simulink model "Simulink_Simulink_PIL_Cruise_Crontrol_r2020b"  (R2024a)
settings: Solver=VariableStepAuto  StartTime=0.0  StopTime=Tsim  FixedStep=Ts/20  RelTol=1e-3
undefined symbols (not defined in the file or in its folder): g, noise, PIL, Ts
libraries: simulink x2, aerolibactuator x1, aerolibatmos2 x1
settings Model: SimulationMode=accelerator  Creator=ricardo  LastModifiedBy=mason
settings SolverCC: AlgebraicLoopSolver=TrustRegion
settings DataIOCC: ReturnWorkspaceOutputs=off
settings DebuggingCC: UnconnectedInputMsg=warning  UnconnectedOutputMsg=warning  UnconnectedLineMsg=warning  ArithmeticOperatorsInVariantConditions=warning
settings ModelReferenceCC: EnableRefExpFcnMdlSchedulingChecks=on
settings SFSimCC: CustomCodeUndefinedFunction=UseInterfaceOnly
settings RTWCC: GPUComputeCapability=3.5  DLArmComputeVersion=19.05

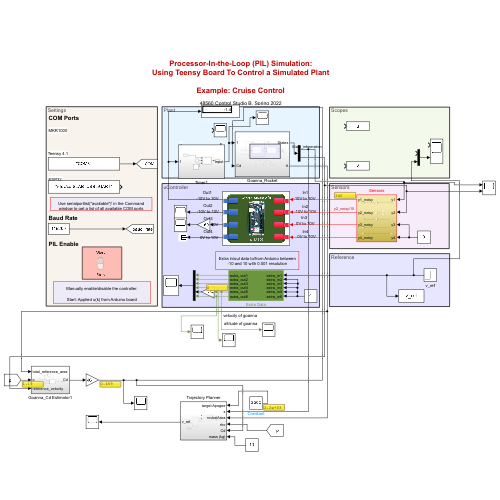
[thumbnail: Simulink's stored preview of the top-level diagram]
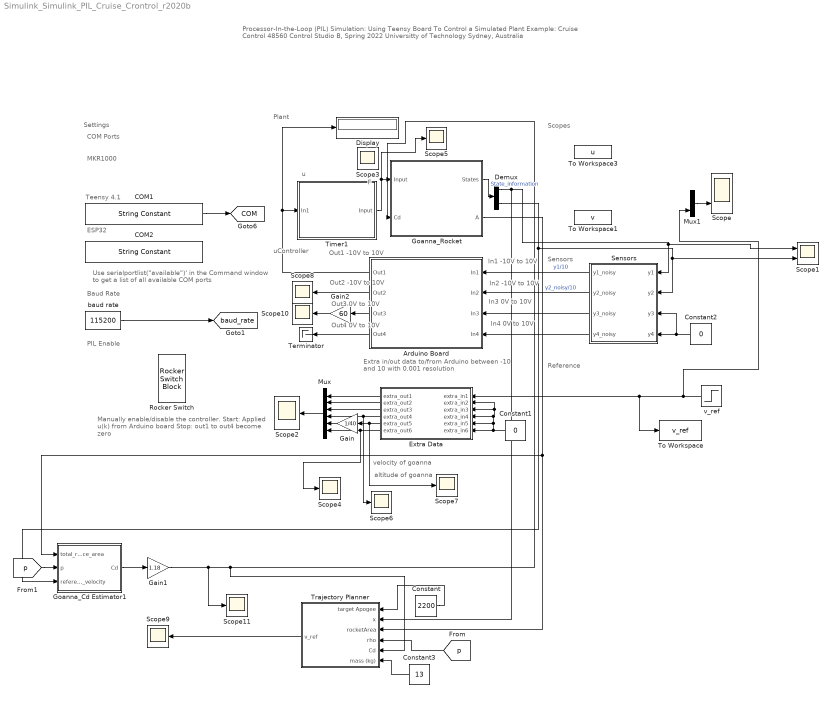
== system Simulink_Simulink_PIL_Cruise_Crontrol_r2020b ==
  note: altitude of goanna
  note: velocity of goanna
  note: F
  note: u
  note: MKR1000
  note: COM Ports
  note: Settings
  note: Scopes
  note: Plant
  note: Reference
  note: Sensors
  note: uController
  note: Out1
      | -10V to 10V
  note: Processor-In-the-Loop (PIL) Simulation:
      | Using Teensy Board To Control a Simulated Plant
      |
      | Example: Cruise Control
      |
      | 48560 Control Studio B, Spring 2022
      | Universitty of Technology Sydney, Australia
  note: Out2
      | -10V to 10V
  note: Out3
      | 0V to 10V
  note: Out4
      | 0V to 10V
  note: In1
      | -10V to 10V
  note: In2
      | -10V to 10V
  note: In3
      | 0V to 10V
  note: In4
      | 0V to 10V
  note: Manually enable/disable the controller.
      |
      | Start: Applied u(k) from Arduino board
      | Stop: out1 to out4 become zero
  note: Extra in/out data to/from Arduino between -10 and 10 with 0.001 resolution
  note: Baud Rate
  note: PIL Enable
  note: Use serialportlist("available")' in the Command window to get a list of all available COM ports
  note: ESP32
  note: Teensy 4.1
  Arduino Board : Subsystem
      mask Display: image('$imagefile'); % Use "Edit Image" on toolstrip to change.
  COM1 : StringConstant  String="\"COM8\""
  COM2 : StringConstant  String="\"/dev/cu.SLAB_USBtoUART\""
  Constant : Constant  Value=2200
  Constant1 : Constant  Value=0
  Constant2 : Constant  Value=0
  Constant3 : Constant  Value=13
  Demux : Demux  Outputs=2
  Display : Display
  Extra Data : Subsystem
  Gain : Gain  Gain=1/40
  Gain1 : Gain  Gain=1.18
  Gain2 : Gain  Gain=60
  Goanna_Cd Estimator1 : Subsystem
  Goanna_Rocket : Subsystem
  Mux : Mux  Inputs=6
  Mux1 : Mux  Inputs=2
  Rocker Switch : RockerSwitchBlock  LabelPosition=Hide
      settings: Values={{'Stop', 'Start'}, [0 1]}
  Scope : Scope  NumInputPorts=2
  Scope1 : Scope  NumInputPorts=2
  Scope{2..11} (10 alike) : Scope
  Sensors : Subsystem
  Terminator : Terminator
  Timer1 : Subsystem
  To Workspace : ToWorkspace  VariableName=v_ref  SampleTime=Ts/20
  To Workspace1 : ToWorkspace  VariableName=v  SampleTime=Ts/20
  To Workspace3 : ToWorkspace  VariableName=u  SampleTime=Ts/20
  Trajectory Planner : Subsystem
  baud rate : Constant  Value=115200
  v_ref : Step  Time=5  After=5  SampleTime=0
  tag scope: COM=global, baud_rate=global
  wires:
  Arduino Board/2(Out2) -> Scope8/1
  Arduino Board/3(Out3) -> Gain2/1
  Arduino Board/4(Out4) -> Terminator/1
  Extra Data/1(extra_out1) -> Mux/1
  Extra Data/2(extra_out2) -> Mux/2
  Extra Data/3(extra_out3) -> Mux/3
  Extra Data/4(extra_out4) -> Scope6/1, Mux/4
  Mux/1 -> Scope2/1
  Extra Data/5(extra_out5) -> Gain/1, Scope7/1
  Extra Data/6(extra_out6) -> Scope4/1, Mux/6
  Constant1/1 -> Extra Data/2(extra_in2), Extra Data/3(extra_in3), Extra Data/4(extra_in4), Extra Data/5(extra_in5), Extra Data/6(extra_in6)
  Sensors/1(y1_noisy) -> Arduino Board/1(In1)  "y1/10"
  Constant2/1 -> Sensors/3(y3), Sensors/4(y4)
  Sensors/4(y4_noisy) -> Arduino Board/4(In4)
  baud rate/1 -> [baud_rate]
  Sensors/2(y2_noisy) -> Arduino Board/2(In2)  "y2_noisy/10"
  Sensors/3(y3_noisy) -> Arduino Board/3(In3)
  v_ref/1 -> Extra Data/1(extra_in1), To Workspace/1, Mux1/2
  Mux1/1 -> Scope/2
  COM1/1 -> [COM]
  Goanna_Rocket/1(States) -> Demux/1  "State_information"
  Demux/1 -> Scope1/1, Sensors/1(y1), Trajectory Planner/2(x)
  Demux/2 -> Goanna_Cd Estimator1/3(reference_velocity), Scope1/2, Sensors/2(y2)
  Goanna_Cd Estimator1/1(Cd) -> Gain1/1
  Gain/1 -> Mux/5
  Gain1/1 -> Scope11/1, Trajectory Planner/5(Cd), Goanna_Rocket/2(Cd)
  Goanna_Rocket/2(A) -> Trajectory Planner/3(rocketArea), Goanna_Cd Estimator1/1(total_reference_area)
  Constant/1 -> Trajectory Planner/1(target Apogee)
  [p] -> Trajectory Planner/4(rho)
  Constant3/1 -> Trajectory Planner/6(mass (kg))
  [p] -> Goanna_Cd Estimator1/2(p)
  Trajectory Planner/1(v_ref) -> Scope9/1
  Gain2/1 -> Scope10/1
  Timer1/1(Input) -> Scope5/1, Goanna_Rocket/1(Input)
  Arduino Board/1(Out1) -> Display/1, Timer1/1(In1)

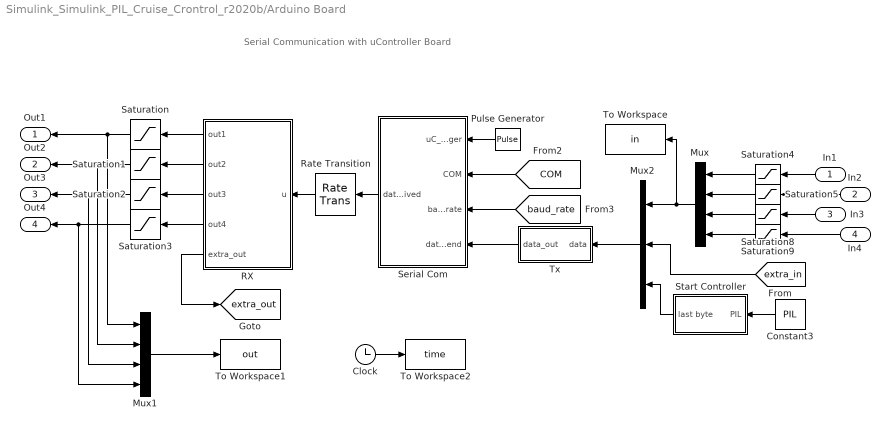
== system Simulink_Simulink_PIL_Cruise_Crontrol_r2020b/Arduino Board ==
  note: Serial Communication with uController Board
  In1 : Inport
  In2 : Inport  Port=2
  In3 : Inport  Port=3
  In4 : Inport  Port=4
  Clock : Clock
  Constant3 : Constant  Value=PIL
  Mux : Mux
  Mux1 : Mux
  Mux2 : Mux  Inputs=3
  Pulse Generator : DiscretePulseGenerator  PulseType=Time based  Period=Ts  PulseWidth=50
  RX : MATLAB Function  TreatAsAtomicUnit=on
  Rate Transition : RateTransition  InitialCondition=zeros(21,1)
  Saturation{,1,4..5} (4 alike) : Saturate  UpperLimit=10  LowerLimit=-10
  Saturation{2..3,8..9} (4 alike) : Saturate  UpperLimit=10  LowerLimit=0
  Serial Com : MATLAB Function  TreatAsAtomicUnit=on  SystemSampleTime=Ts/10
  Start Controller : Subsystem
  To Workspace : ToWorkspace  VariableName=in  SampleTime=Ts/20
  To Workspace1 : ToWorkspace  VariableName=out  SampleTime=Ts/20
  To Workspace2 : ToWorkspace  VariableName=time  SampleTime=Ts/20
  Tx : MATLAB Function  TreatAsAtomicUnit=on  SystemSampleTime=Ts/10
  Out1 : Outport  VectorParamsAs1DForOutWhenUnconnected=off
  Out2 : Outport  Port=2  VectorParamsAs1DForOutWhenUnconnected=off
  Out3 : Outport  Port=3  VectorParamsAs1DForOutWhenUnconnected=off
  Out4 : Outport  Port=4  VectorParamsAs1DForOutWhenUnconnected=off
  tag scope: extra_out=global
  wires:
  RX/1(out1) -> Saturation/1
  RX/2(out2) -> Saturation1/1
  RX/3(out3) -> Saturation2/1
  Mux1/1 -> To Workspace1/1
  Clock/1 -> To Workspace2/1
  Saturation/1 -> Out1/1, Mux1/1
  Saturation1/1 -> Out2/1, Mux1/2
  Saturation2/1 -> Out3/1, Mux1/3
  Saturation3/1 -> Out4/1, Mux1/4
  RX/4(out4) -> Saturation3/1
  RX/5(extra_out) -> [extra_out]
  Mux/1 -> Mux2/1, To Workspace/1
  [COM] -> Serial Com/2(COM)
  [baud_rate] -> Serial Com/3(baud_rate)
  Pulse Generator/1 -> Serial Com/1(uC_trigger)
  Serial Com/1(data_received) -> Rate Transition/1
  Rate Transition/1 -> RX/1(u)
  Constant3/1 -> Start Controller/1(PIL)
  In1/1 -> Saturation4/1
  In2/1 -> Saturation5/1
  In3/1 -> Saturation8/1
  In4/1 -> Saturation9/1
  Saturation4/1 -> Mux/1
  Saturation5/1 -> Mux/2
  Saturation8/1 -> Mux/3
  Saturation9/1 -> Mux/4
  [extra_in] -> Mux2/2
  Start Controller/1(last byte) -> Mux2/3
  Mux2/1 -> Tx/1(data)
  Tx/1(data_out) -> Serial Com/4(data_send)

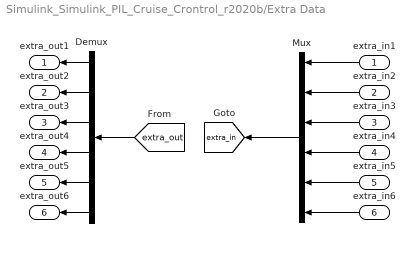
== system Simulink_Simulink_PIL_Cruise_Crontrol_r2020b/Extra Data ==
  extra_in1 : Inport
  extra_in2 : Inport  Port=2
  extra_in3 : Inport  Port=3
  extra_in4 : Inport  Port=4
  extra_in5 : Inport  Port=5
  extra_in6 : Inport  Port=6
  Demux : Demux  Outputs=6
  Mux : Mux  Inputs=6
  extra_out1 : Outport
  extra_out2 : Outport  Port=2
  extra_out3 : Outport  Port=3
  extra_out4 : Outport  Port=4
  extra_out5 : Outport  Port=5
  extra_out6 : Outport  Port=6
  tag scope: extra_in=global
  wires:
  extra_in4/1 -> Mux/4
  extra_in3/1 -> Mux/3
  extra_in2/1 -> Mux/2
  extra_in1/1 -> Mux/1
  Mux/1 -> [extra_in]
  [extra_out] -> Demux/1
  Demux/1 -> extra_out1/1
  Demux/2 -> extra_out2/1
  Demux/3 -> extra_out3/1
  Demux/4 -> extra_out4/1
  extra_in5/1 -> Mux/5
  extra_in6/1 -> Mux/6
  Demux/6 -> extra_out6/1
  Demux/5 -> extra_out5/1

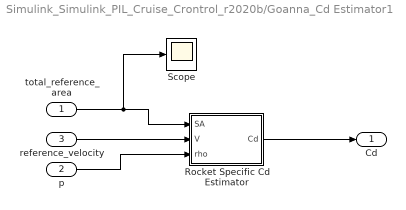
== system Simulink_Simulink_PIL_Cruise_Crontrol_r2020b/Goanna_Cd Estimator1 ==
  total_reference_area : Inport
  p : Inport  Port=2
  reference_velocity : Inport  Port=3
  Rocket Specific Cd Estimator : MATLAB Function  TreatAsAtomicUnit=on
  Scope : Scope
  Cd : Outport
  wires:
  Rocket Specific Cd Estimator/1(Cd) -> Cd/1
  total_reference_area/1 -> Scope/1, Rocket Specific Cd Estimator/1(SA)
  reference_velocity/1 -> Rocket Specific Cd Estimator/2(V)
  p/1 -> Rocket Specific Cd Estimator/3(rho)

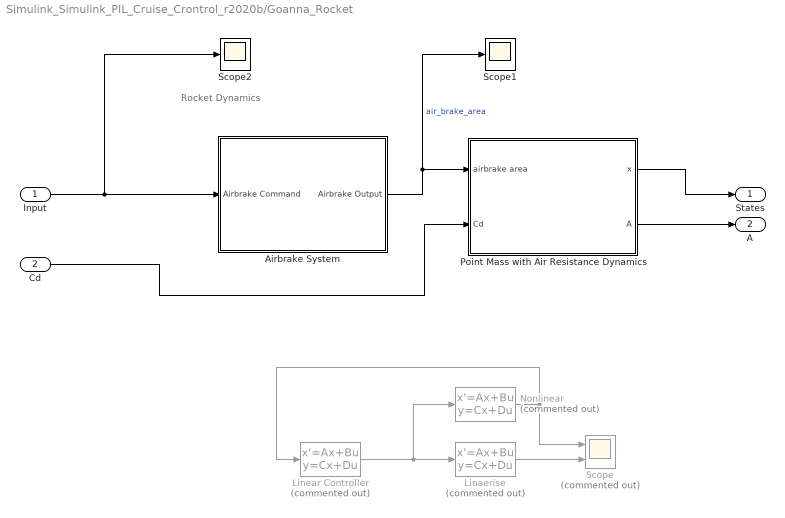
== system Simulink_Simulink_PIL_Cruise_Crontrol_r2020b/Goanna_Rocket ==
  note: Rocket Dynamics
  Input : Inport
  Cd : Inport  Port=2
  Airbrake System : Subsystem
      mask Display: image('airbrake.png');
  "Linaerise " : StateSpace  Commented=on  InitialCondition=0
  Linear Controller : StateSpace  Commented=on  InitialCondition=0
  Nonlinear : StateSpace  Commented=on  InitialCondition=0
  "Point Mass with Air Resistance Dynamics " : Subsystem
      mask Display: image('rocket.jpeg');
  Scope : Scope  Commented=on  NumInputPorts=2
  Scope1 : Scope
  Scope2 : Scope
  States : Outport
  A : Outport  Port=2
  wires:
  "Point Mass with Air Resistance Dynamics "/1(x) -> States/1
  Linear Controller/1 -> Nonlinear/1, "Linaerise "/1
  Nonlinear/1 -> Linear Controller/1, Scope/1
  "Linaerise "/1 -> Scope/2
  Input/1 -> Scope2/1, Airbrake System/1(Airbrake Command)
  Airbrake System/1(Airbrake Output) -> "Point Mass with Air Resistance Dynamics "/1(airbrake area), Scope1/1  "air_brake_area"
  Cd/1 -> "Point Mass with Air Resistance Dynamics "/2(Cd)
  "Point Mass with Air Resistance Dynamics "/2(A) -> A/1

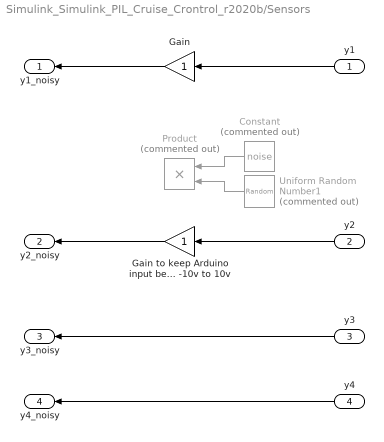
== system Simulink_Simulink_PIL_Cruise_Crontrol_r2020b/Sensors ==
  y1 : Inport
  y2 : Inport  Port=2
  y3 : Inport  Port=3
  y4 : Inport  Port=4
  Constant : Constant  Commented=on  Value=noise
  Gain : Gain
  "Gain to keep Arduino input between -10v to 10v " : Gain
  Product : Product  Commented=on
  Uniform Random Number1 : UniformRandomNumber  Commented=on  Minimum=-0.1  Maximum=0.1  SampleTime=0.5*Ts
  y1_noisy : Outport  VectorParamsAs1DForOutWhenUnconnected=off
  y2_noisy : Outport  Port=2  VectorParamsAs1DForOutWhenUnconnected=off
  y3_noisy : Outport  Port=3  VectorParamsAs1DForOutWhenUnconnected=off
  y4_noisy : Outport  Port=4  VectorParamsAs1DForOutWhenUnconnected=off
  wires:
  y2/1 -> "Gain to keep Arduino input between -10v to 10v "/1
  y3/1 -> y3_noisy/1
  y4/1 -> y4_noisy/1
  y1/1 -> Gain/1
  Uniform Random Number1/1 -> Product/2
  Constant/1 -> Product/1
  "Gain to keep Arduino input between -10v to 10v "/1 -> y2_noisy/1
  Gain/1 -> y1_noisy/1

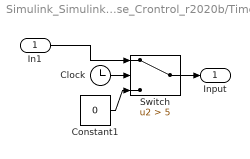
== system Simulink_Simulink_PIL_Cruise_Crontrol_r2020b/Timer1 ==
  In1 : Inport
  Clock : Clock
  Constant1 : Constant  Value=0
  Switch : Switch  Criteria=u2 > Threshold  Threshold=5  SaturateOnIntegerOverflow=off  InputSameDT=off
  Input : Outport
  wires:
  Switch/1 -> Input/1
  Clock/1 -> Switch/2
  In1/1 -> Switch/1
  Constant1/1 -> Switch/3

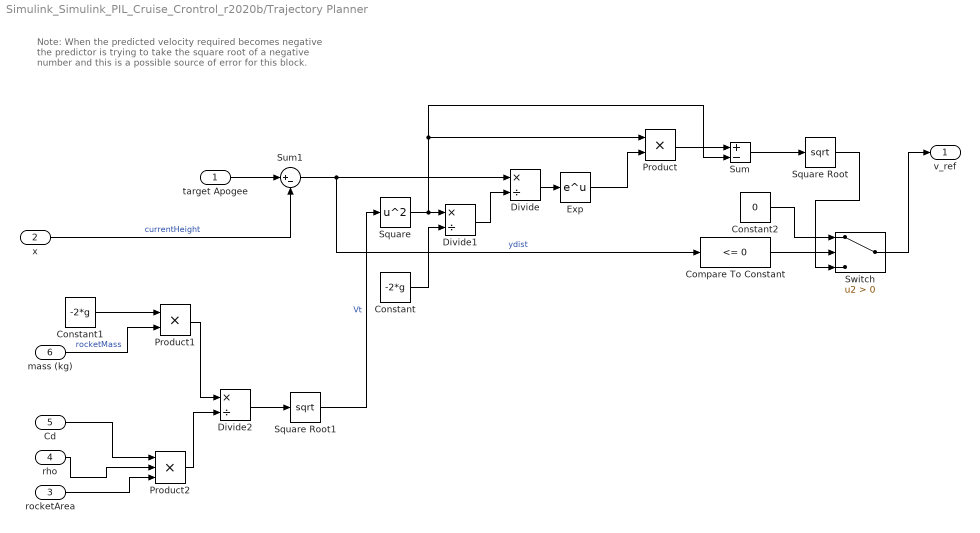
== system Simulink_Simulink_PIL_Cruise_Crontrol_r2020b/Trajectory Planner ==
  note: Note: When the predicted velocity required becomes negative the predictor is trying to take the square root of a negative number and this is a possible source of error for this block.
  target Apogee : Inport
  x : Inport  Port=2
  rocketArea : Inport  Port=3
  rho : Inport  Port=4
  Cd : Inport  Port=5
  mass (kg) : Inport  Port=6
  Compare To Constant : simulink/Logic and Bit Operations/Compare To Constant  relop=<=  const=0  OutDataTypeStr=boolean
  Constant : Constant  Value=-2*g
  Constant1 : Constant  Value=-2*g
  Constant2 : Constant  Value=0
  Divide : Product  Inputs=*/
  Divide1 : Product  Inputs=*/
  Divide2 : Product  Inputs=*/
  Exp : Math
  Product : Product
  Product1 : Product
  Product2 : Product  Inputs=3
  Square : Math  Operator=square
  Square Root : Sqrt
  Square Root1 : Sqrt
  Sum : Sum  Inputs=+-
  Sum1 : Sum  Inputs=|+-
  Switch : Switch  Criteria=u2 > Threshold  SaturateOnIntegerOverflow=off  InputSameDT=off
  v_ref : Outport
  wires:
  Sum/1 -> Square Root/1
  Product/1 -> Sum/1
  Exp/1 -> Product/2
  Divide/1 -> Exp/1
  Sum1/1 -> Compare To Constant/1, Divide/1  "ydist"
  Constant/1 -> Divide1/2
  Divide1/1 -> Divide/2
  Square/1 -> Sum/2, Product/1, Divide1/1
  target Apogee/1 -> Sum1/1
  Product2/1 -> Divide2/2
  Square Root1/1 -> Square/1  "Vt"
  Cd/1 -> Product2/1
  Divide2/1 -> Square Root1/1
  rocketArea/1 -> Product2/3
  Product1/1 -> Divide2/1
  Constant1/1 -> Product1/1
  rho/1 -> Product2/2
  mass (kg)/1 -> Product1/2  "rocketMass"
  x/1 -> Sum1/2  "currentHeight"
  Compare To Constant/1 -> Switch/2
  Constant2/1 -> Switch/1
  Square Root/1 -> Switch/3
  Switch/1 -> v_ref/1

== system Simulink_Simulink_PIL_Cruise_Crontrol_r2020b/Arduino Board/Start Controller ==
  PIL : Inport
  Constant : Constant  Value=0
  Constant1 : Constant  Value=255
  Switch : Switch  Criteria=u2 > Threshold  SaturateOnIntegerOverflow=off  InputSameDT=off
  last byte : Outport
  wires:
  Switch/1 -> last byte/1
  PIL/1 -> Switch/2
  Constant1/1 -> Switch/1
  Constant/1 -> Switch/3

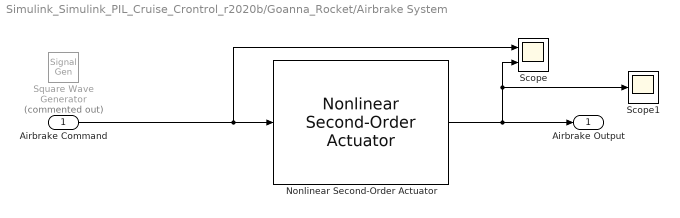
== system Simulink_Simulink_PIL_Cruise_Crontrol_r2020b/Goanna_Rocket/Airbrake System ==
  Airbrake Command : Inport
  Nonlinear Second-Order Actuator : aerolibactuator/Nonlinear Second-Order Actuator  wn_fin=10  z_fin=0.7  fin_max=maxAirbrakeArea  fin_min=0  fin_maxrate=0.4  fin_act_0=0  fin_act_vel=0
  Scope : Scope  NumInputPorts=2
  Scope1 : Scope
  Square Wave Generator : SignalGenerator  Commented=on  WaveForm=square  Amplitude=0.01  Units=rad/sec
  Airbrake Output : Outport
  wires:
  Nonlinear Second-Order Actuator/1 -> Scope1/1, Scope/2, Airbrake Output/1
  Airbrake Command/1 -> Nonlinear Second-Order Actuator/1, Scope/1

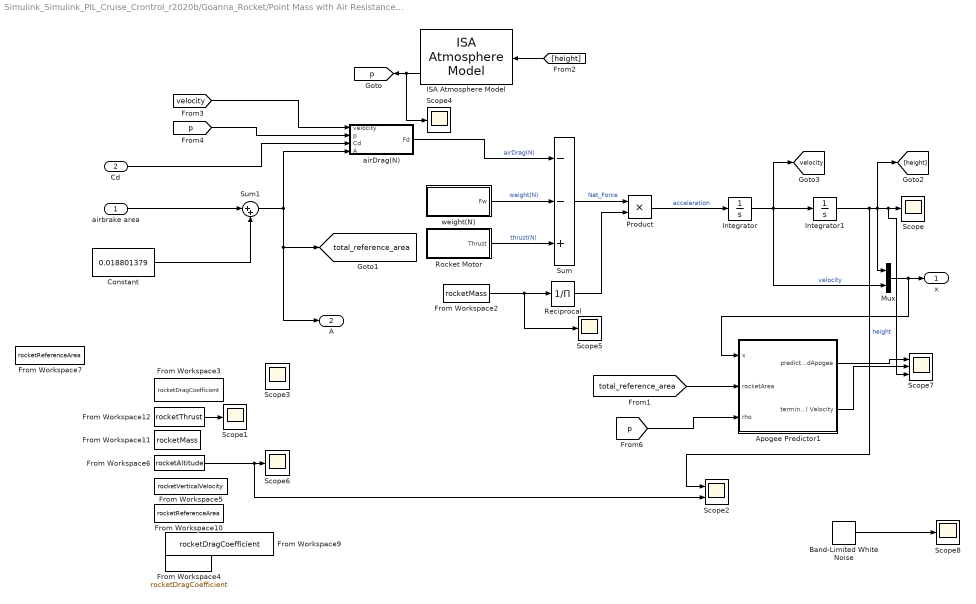
== system Simulink_Simulink_PIL_Cruise_Crontrol_r2020b/Goanna_Rocket/Point Mass with Air Resistance Dynamics  ==
  airbrake area : Inport
  Cd : Inport  Port=2
  Apogee Predictor1 : Subsystem
  Band-Limited White Noise : simulink/Sources/Band-Limited White Noise  Cov=[0.1]  Ts=0.1  seed=[23341]
  Constant : Constant  Value=0.018801379
  From Workspace10 : FromWorkspace  VariableName=rocketReferenceArea
  From Workspace11 : FromWorkspace  VariableName=rocketMass
  From Workspace12 : FromWorkspace  VariableName=rocketThrust
  From Workspace2 : FromWorkspace  VariableName=rocketMass
  From Workspace3 : FromWorkspace  VariableName=rocketDragCoefficient
  From Workspace4 : FromWorkspace  VariableName=rocketDragCoefficient
  From Workspace5 : FromWorkspace  VariableName=rocketVerticalVelocity
  From Workspace6 : FromWorkspace  VariableName=rocketAltitude
  From Workspace7 : FromWorkspace  VariableName=rocketReferenceArea
  From Workspace9 : FromWorkspace  VariableName=rocketDragCoefficient
  ISA Atmosphere Model : aerolibatmos2/ISA Atmosphere Model  useExtended=off  action=Warning  custom=on  viscosityOut=off  g=9.80665  gamma=1.4  R=287.0531  L=0.0065  h_trop=11000  h_strat=20000  rho0=1.225  P0=101325  T0=288.15  h0=0  S=110.4  Tref=273.15  muref=1.716e-5
  Integrator : Integrator
  Integrator1 : Integrator
  Mux : Mux  Inputs=2
  Product : Product
  Reciprocal : Product  Inputs=/
  "Rocket Motor " : Subsystem
  Scope{,1,4..6,8} (6 alike) : Scope
  Scope2 : Scope  NumInputPorts=2
  Scope3 : Scope  NumInputPorts=2
  Scope7 : Scope  NumInputPorts=3
  Sum : Sum  Inputs=--+
  Sum1 : Sum  Inputs=|++
  airDrag(N) : Subsystem
  weight(N) : Subsystem
  x : Outport
  A : Outport  Port=2
  tag scope: p=global, total_reference_area=global, velocity=global
  wires:
  "Rocket Motor "/1(Thrust) -> Sum/3  "thrust(N)"
  weight(N)/1(Fw) -> Sum/2  "weight(N)"
  Sum/1 -> Product/1  "Net_Force"
  ISA Atmosphere Model/4 -> Scope4/1, [p]
  [height] -> ISA Atmosphere Model/1
  [velocity] -> airDrag(N)/1(velocity)
  [p] -> airDrag(N)/2(p)
  Product/1 -> Integrator/1  "acceleration"
  Integrator/1 -> [velocity], Integrator1/1, Mux/2  "velocity"
  Integrator1/1 -> Scope2/1, Mux/1, [height], Scope7/3, Scope/1  "height"
  Mux/1 -> Apogee Predictor1/1(x), x/1
  Reciprocal/1 -> Product/2
  From Workspace2/1 -> Scope5/1, Reciprocal/1
  From Workspace12/1 -> Scope1/1
  airbrake area/1 -> Sum1/1
  Sum1/1 -> A/1, [total_reference_area], airDrag(N)/4(A)
  Constant/1 -> Sum1/2
  airDrag(N)/1(Fd) -> Sum/1  "airDrag(N)"
  From Workspace6/1 -> Scope2/2, Scope6/1
  [total_reference_area] -> Apogee Predictor1/2(rocketArea)
  [p] -> Apogee Predictor1/3(rho)
  Apogee Predictor1/1(predictedApogee) -> Scope7/1
  Apogee Predictor1/2(terminal Velocity) -> Scope7/2
  Band-Limited White Noise/1 -> Scope8/1
  Cd/1 -> airDrag(N)/3(Cd)

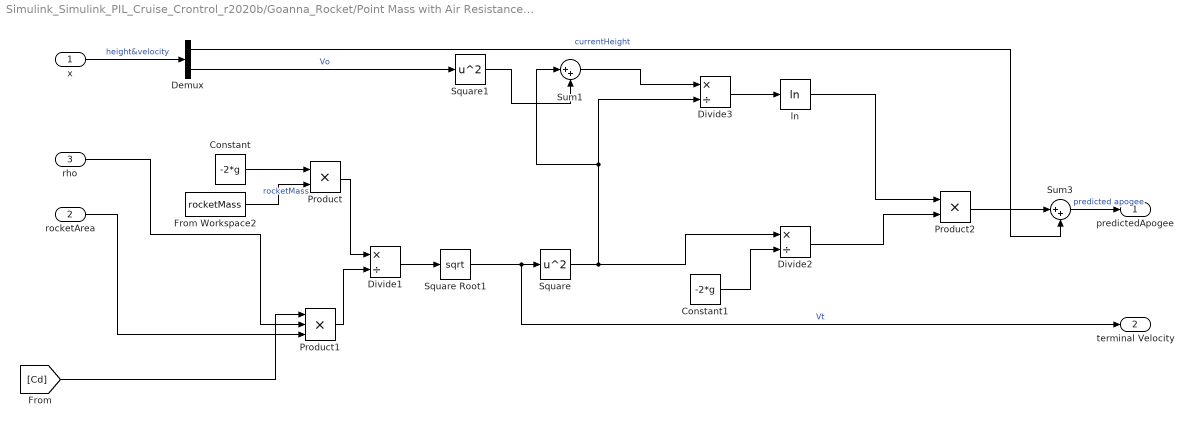
== system Simulink_Simulink_PIL_Cruise_Crontrol_r2020b/Goanna_Rocket/Point Mass with Air Resistance Dynamics /Apogee Predictor1 ==
  x : Inport
  rocketArea : Inport  Port=2
  rho : Inport  Port=3
  Constant : Constant  Value=-2*g
  Constant1 : Constant  Value=-2*g
  Demux : Demux  Outputs=2
  Divide1 : Product  Inputs=*/
  Divide2 : Product  Inputs=*/
  Divide3 : Product  Inputs=*/
  From Workspace2 : FromWorkspace  VariableName=rocketMass
  Product : Product
  Product1 : Product  Inputs=3
  Product2 : Product
  Square : Math  Operator=square
  Square Root1 : Sqrt
  Square1 : Math  Operator=square
  Sum1 : Sum  Inputs=|++
  Sum3 : Sum  Inputs=|++
  ln : Math  Operator=log
  predictedApogee : Outport
  terminal Velocity : Outport  Port=2
  wires:
  Constant/1 -> Product/1
  Product/1 -> Divide1/1
  Product1/1 -> Divide1/2
  [Cd] -> Product1/1
  rho/1 -> Product1/2
  rocketArea/1 -> Product1/3
  Divide1/1 -> Square Root1/1
  Square Root1/1 -> terminal Velocity/1, Square/1  "Vt"
  Product2/1 -> Sum3/1
  ln/1 -> Product2/1
  Divide2/1 -> Product2/2
  Square/1 -> Divide3/2, Sum1/1, Divide2/1
  Constant1/1 -> Divide2/2
  Divide3/1 -> ln/1
  Square1/1 -> Sum1/2
  Sum1/1 -> Divide3/1
  x/1 -> Demux/1  "height&velocity"
  From Workspace2/1 -> Product/2  "rocketMass"
  Demux/2 -> Square1/1  "Vo"
  Demux/1 -> Sum3/2  "currentHeight"
  Sum3/1 -> predictedApogee/1  "predicted apogee"

== system Simulink_Simulink_PIL_Cruise_Crontrol_r2020b/Goanna_Rocket/Point Mass with Air Resistance Dynamics /Rocket Motor  ==
  From Workspace12 : FromWorkspace  VariableName=rocketThrust
  Gain : Gain  Gain=1.0
  Thrust : Outport
  wires:
  From Workspace12/1 -> Gain/1
  Gain/1 -> Thrust/1

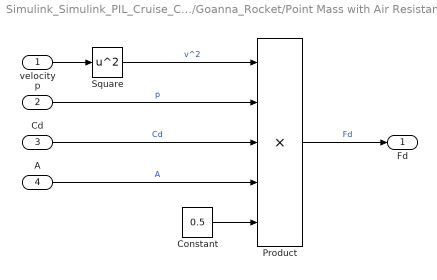
== system Simulink_Simulink_PIL_Cruise_Crontrol_r2020b/Goanna_Rocket/Point Mass with Air Resistance Dynamics /airDrag(N) ==
  velocity : Inport
  p : Inport  Port=2
  Cd : Inport  Port=3
  A : Inport  Port=4
  Constant : Constant  Value=0.5
  Product : Product  Inputs=5
  Square : Math  Operator=square
  Fd : Outport
  wires:
  velocity/1 -> Square/1
  Square/1 -> Product/1  "v^2"
  p/1 -> Product/2  "p"
  Cd/1 -> Product/3  "Cd"
  A/1 -> Product/4  "A"
  Constant/1 -> Product/5
  Product/1 -> Fd/1  "Fd"

== system Simulink_Simulink_PIL_Cruise_Crontrol_r2020b/Goanna_Rocket/Point Mass with Air Resistance Dynamics /weight(N) ==
  From Workspace11 : FromWorkspace  VariableName=rocketMass
  gravity : Gain  Gain=9.80665
  Fw : Outport
  wires:
  From Workspace11/1 -> gravity/1
  gravity/1 -> Fw/1

== matlab function Simulink_Simulink_PIL_Cruise_Crontrol_r2020b/Arduino Board/RX ==
  data: u input; out1 output; out2 output; out3 output; out4 output; extra_out output
%% Rx Data from uController Board
% 
%
% Control Studio A/B,
% The University of Technology Sydney (UTS)
% Sydney, NSW, Australia
%
% Dr Ricardo P. Aguilera
% August 2021
%%%%%%%%%%%%%%%%%%%%%%%%%%%%%%%%%%%%%%%%%%%%%%%%%%%%%%%%%%%%%%%%%%%%%%%%%%%%

function [out1, out2, out3, out4, extra_out] = fcn(u)
    [out1, out2, out3, out4, extra_out] = uC_Rx(u);
end

== matlab function Simulink_Simulink_PIL_Cruise_Crontrol_r2020b/Arduino Board/Serial Com ==
  data: uC_trigger input; COM input; baud_rate input; data_received output; data_send input
%% Serial Communicaiton to/from uController Board
% 
%
% Control Studio A/B,
% The University of Technology Sydney (UTS)
% Sydney, NSW, Australia
%
% Dr Ricardo P. Aguilera
% August 2021
%%%%%%%%%%%%%%%%%%%%%%%%%%%%%%%%%%%%%%%%%%%%%%%%%%%%%%%%%%%%%%%%%%%%%%%%%%%%

function data_received  = fcn(uC_trigger, COM, baud_rate, data_send)
    data_received = uC_SerialCom(uC_trigger, COM, baud_rate, data_send);
end

== matlab function Simulink_Simulink_PIL_Cruise_Crontrol_r2020b/Arduino Board/Tx ==
  data: data input; data_out output
%% Data preconditioning to be sent to uController Board
% 
%
% Control Studio A/B,
% The University of Technology Sydney (UTS)
% Sydney, NSW, Australia
%
% Dr Ricardo P. Aguilera
% August 2021
%%%%%%%%%%%%%%%%%%%%%%%%%%%%%%%%%%%%%%%%%%%%%%%%%%%%%%%%%%%%%%%%%%%%%%%%%%%%
function data_out = fcn(data)
    data_out = uC_Tx(data);
end

== matlab function Simulink_Simulink_PIL_Cruise_Crontrol_r2020b/Goanna_Cd Estimator1/Rocket Specific Cd Estimator ==
  data: SA input; Cd output; V input; rho input
function Cd = fcn(SA,V,rho)
u1 =  21.038140859140483;  % Total rocket SA.
u2 = -0.00013081819610389527; % Velocity
u3 = -0.01571134830357142; % Air density
intercept = -0.008812382900499849;
Cd = (SA*u1)+ (V*u2)+ (rho*u3) + (intercept) ;
end
